simulink model "soru1f"  (R2019a)
settings: Solver=VariableStepAuto  StartTime=0.0  StopTime=100  RelTol=1e-3
libraries: simulink x1
settings Model: Creator=handeyildirim  LastModifiedBy=handeyildirim

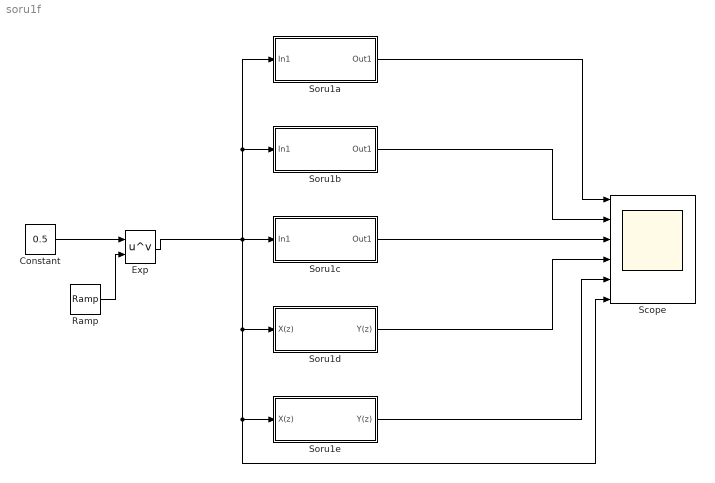
== system soru1f ==
  Constant : Constant  Value=0.5
  Exp : Math  Operator=pow  OutputSignalType=real  OutMin=0  SaturateOnIntegerOverflow=on
  Ramp : simulink/Sources/Ramp  slope=1  start=0  InitialOutput=0
  Scope : Scope  NumInputPorts=6
  Soru1a : Subsystem
  Soru1b : Subsystem
  Soru1c : Subsystem
  Soru1d : Subsystem
  Soru1e : Subsystem
  wires:
  Exp/1 -> Soru1a/1(In1), Soru1b/1(In1), Soru1d/1(X(z)), Soru1e/1(X(z)), Scope/6, Soru1c/1(In1)
  Soru1a/1(Out1) -> Scope/1
  Soru1b/1(Out1) -> Scope/2
  Soru1c/1(Out1) -> Scope/3
  Soru1d/1(Y(z)) -> Scope/4
  Soru1e/1(Y(z)) -> Scope/5
  Constant/1 -> Exp/1
  Ramp/1 -> Exp/2

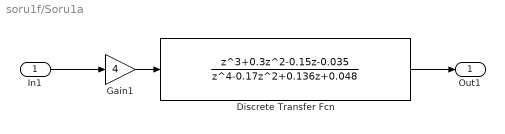
== system soru1f/Soru1a ==
  In1 : Inport
  Discrete Transfer Fcn : DiscreteTransferFcn  Numerator=[1 0.3 -0.15 -0.035]  Denominator=[1 0 -0.17 0.136 0.048]  SampleTime=1
  Gain1 : Gain  Gain=4
  Out1 : Outport
  wires:
  Gain1/1 -> Discrete Transfer Fcn/1
  Discrete Transfer Fcn/1 -> Out1/1
  In1/1 -> Gain1/1

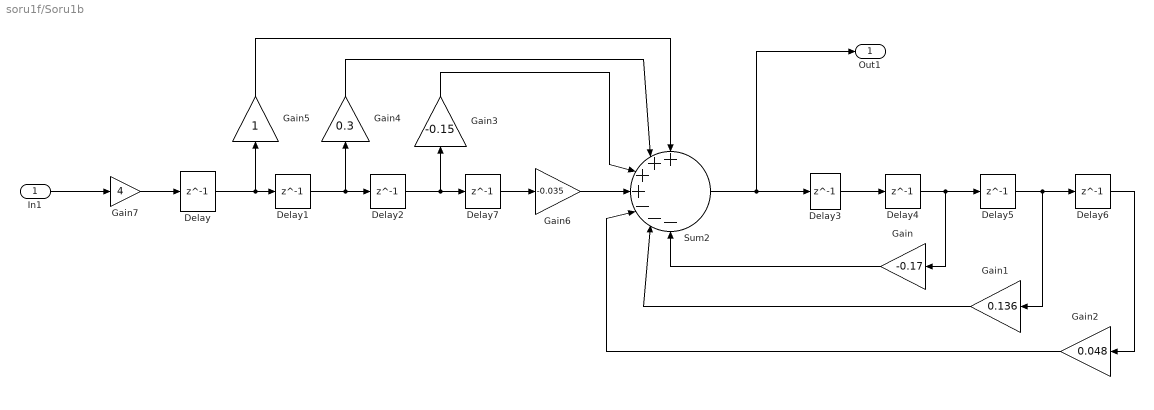
== system soru1f/Soru1b ==
  In1 : Inport
  Delay{,1..7} (8 alike) : Delay  DelayLength=1
  Gain : Gain  Gain=-0.17
  Gain1 : Gain  Gain=0.136
  Gain2 : Gain  Gain=0.048
  Gain3 : Gain  Gain=-0.15
  Gain4 : Gain  Gain=0.3
  Gain5 : Gain
  Gain6 : Gain  Gain=-0.035
  Gain7 : Gain  Gain=4
  Sum2 : Sum  Inputs=++++---
  Out1 : Outport
  wires:
  Delay/1 -> Delay1/1, Gain5/1
  Gain/1 -> Sum2/7
  Gain2/1 -> Sum2/5
  Delay1/1 -> Delay2/1, Gain4/1
  In1/1 -> Gain7/1
  Delay6/1 -> Gain2/1
  Sum2/1 -> Out1/1, Delay3/1
  Delay7/1 -> Gain6/1
  Gain6/1 -> Sum2/4
  Delay5/1 -> Gain1/1, Delay6/1
  Gain5/1 -> Sum2/1
  Delay4/1 -> Gain/1, Delay5/1
  Delay3/1 -> Delay4/1
  Delay2/1 -> Delay7/1, Gain3/1
  Gain4/1 -> Sum2/2
  Gain3/1 -> Sum2/3
  Gain7/1 -> Delay/1
  Gain1/1 -> Sum2/6

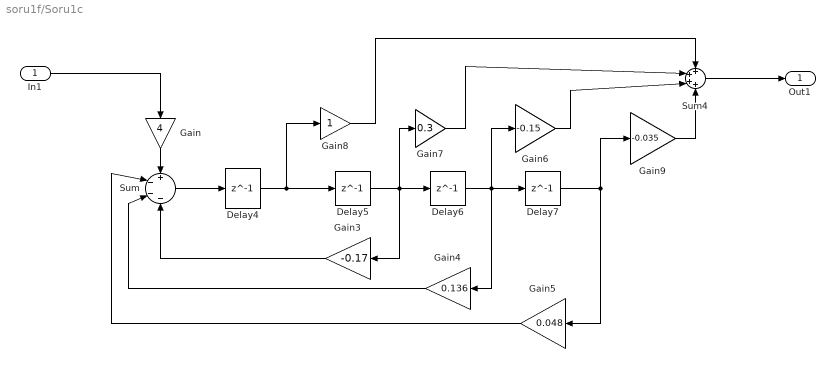
== system soru1f/Soru1c ==
  In1 : Inport
  Delay{4..7} (4 alike) : Delay  DelayLength=1
  Gain : Gain  Gain=4
  Gain3 : Gain  Gain=-0.17
  Gain4 : Gain  Gain=0.136
  Gain5 : Gain  Gain=0.048
  Gain6 : Gain  Gain=-0.15
  Gain7 : Gain  Gain=0.3
  Gain8 : Gain
  Gain9 : Gain  Gain=-0.035
  Sum : Sum  Inputs=+---
  Sum4 : Sum  Inputs=++++
  Out1 : Outport
  wires:
  Gain/1 -> Sum/1
  In1/1 -> Gain/1
  Gain9/1 -> Sum4/4
  Gain3/1 -> Sum/4
  Sum/1 -> Delay4/1
  Gain5/1 -> Sum/2
  Gain7/1 -> Sum4/2
  Gain6/1 -> Sum4/3
  Delay6/1 -> Delay7/1, Gain4/1, Gain6/1
  Delay5/1 -> Delay6/1, Gain3/1, Gain7/1
  Delay7/1 -> Gain5/1, Gain9/1
  Gain4/1 -> Sum/3
  Gain8/1 -> Sum4/1
  Delay4/1 -> Delay5/1, Gain8/1
  Sum4/1 -> Out1/1

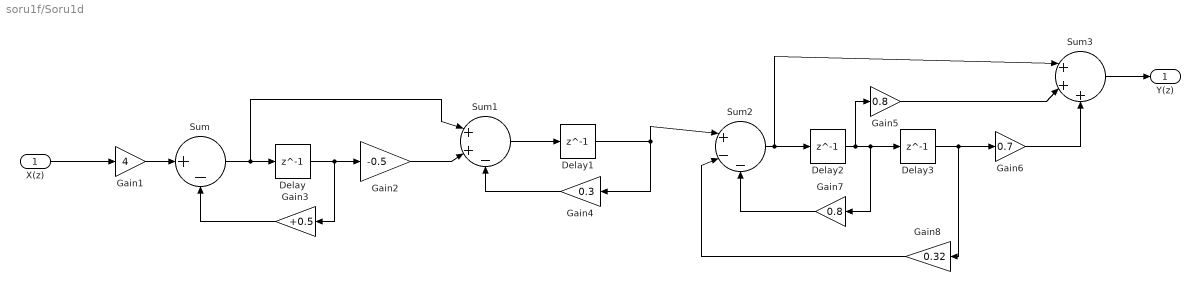
== system soru1f/Soru1d ==
  X(z) : Inport
  Delay{,1..3} (4 alike) : Delay  DelayLength=1
  Gain1 : Gain  Gain=4
  Gain2 : Gain  Gain=-0.5
  Gain3 : Gain  Gain=+0.5
  Gain4 : Gain  Gain=0.3
  Gain5 : Gain  Gain=0.8
  Gain6 : Gain  Gain=0.7
  Gain7 : Gain  Gain=0.8
  Gain8 : Gain  Gain=0.32
  Sum : Sum  Inputs=|+-
  Sum1 : Sum  Inputs=|++-
  Sum2 : Sum  Inputs=|+--
  Sum3 : Sum  Inputs=|+++
  Y(z) : Outport
  wires:
  Gain1/1 -> Sum/1
  Sum3/1 -> Y(z)/1
  Gain2/1 -> Sum1/2
  Gain7/1 -> Sum2/3
  Gain3/1 -> Sum/2
  Gain4/1 -> Sum1/3
  Sum/1 -> Delay/1, Sum1/1
  X(z)/1 -> Gain1/1
  Delay3/1 -> Gain8/1, Gain6/1
  Sum2/1 -> Delay2/1, Sum3/1
  Delay/1 -> Gain3/1, Gain2/1
  Delay1/1 -> Gain4/1, Sum2/1
  Gain5/1 -> Sum3/2
  Delay2/1 -> Gain5/1, Gain7/1, Delay3/1
  Gain6/1 -> Sum3/3
  Sum1/1 -> Delay1/1
  Gain8/1 -> Sum2/2

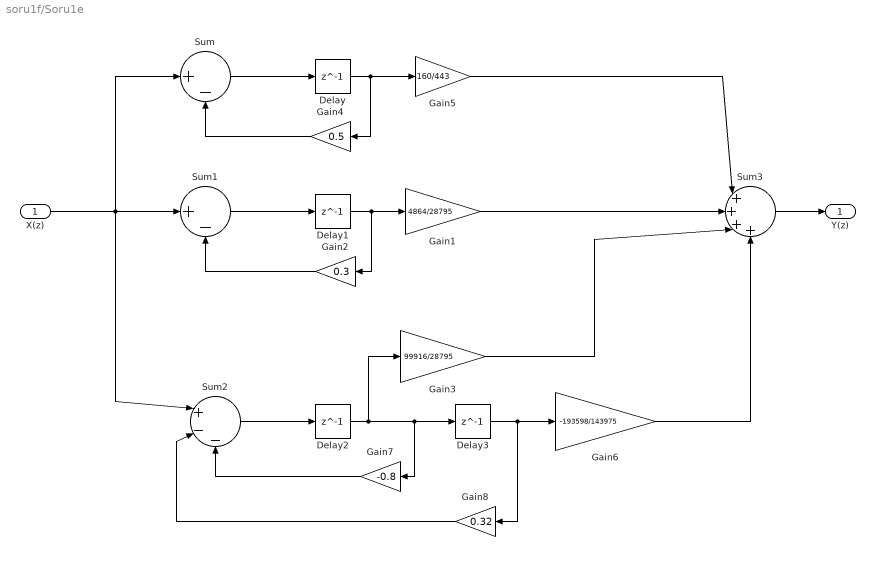
== system soru1f/Soru1e ==
  X(z) : Inport
  Delay{,1..3} (4 alike) : Delay  DelayLength=1
  Gain1 : Gain  Gain=4864/28795
  Gain2 : Gain  Gain=0.3
  Gain3 : Gain  Gain=99916/28795
  Gain4 : Gain  Gain=0.5
  Gain5 : Gain  Gain=160/443
  Gain6 : Gain  Gain=-193598/143975
  Gain7 : Gain  Gain=-0.8
  Gain8 : Gain  Gain=0.32
  Sum : Sum  Inputs=|+-
  Sum1 : Sum  Inputs=|+-
  Sum2 : Sum  Inputs=|+--
  Sum3 : Sum  Inputs=|++++
  Y(z) : Outport
  wires:
  Gain1/1 -> Sum3/2
  Gain4/1 -> Sum/2
  Gain7/1 -> Sum2/3
  Delay1/1 -> Gain2/1, Gain1/1
  Sum3/1 -> Y(z)/1
  Sum1/1 -> Delay1/1
  Gain6/1 -> Sum3/4
  Sum2/1 -> Delay2/1
  Gain5/1 -> Sum3/1
  Delay/1 -> Gain4/1, Gain5/1
  Sum/1 -> Delay/1
  Delay2/1 -> Gain3/1, Gain7/1, Delay3/1
  Gain2/1 -> Sum1/2
  Delay3/1 -> Gain8/1, Gain6/1
  Gain3/1 -> Sum3/3
  Gain8/1 -> Sum2/2
  X(z)/1 -> Sum1/1, Sum/1, Sum2/1
